simulink model "RRR_with_CTC_task_space"  (Simulink 8.5)
settings: Solver=ode113  StartTime=0.0  StopTime=T_f  RelTol=RT  AbsTol=AT
values from neighbouring files (symbols this model uses):
  kp = x(24)    [PRBDM_3R_CTC.m]    (also in PRBDM_3R_main.m = 20; PRBDM_3R_test001.m = 2; PRBDM_CTC_task.m = z(30); RRR_CTC.m)
  kv = x(23)    [PRBDM_3R_CTC.m]    (also in PRBDM_3R_main.m = 40; PRBDM_3R_test001.m = 4; PRBDM_CTC_task.m = z(29); RRR_CTC.m)
  L1 = z(8)    [Forward_kinematics.m]    (also in GeometricCalculation_simulink.m = Geoparams(5); Jacobi.m = x(4); PRBDM_3R_CTC.m = x(19); PRBDM_3R_Dynamic_Matrices_NewtonEular.m = robot_params(4))
  L2 = z(9)    [Forward_kinematics.m]    (also in GeometricCalculation_simulink.m = Geoparams(6); Jacobi.m = x(5); PRBDM_3R_CTC.m = x(20); PRBDM_3R_Dynamic_Matrices_NewtonEular.m = robot_params(5))
  L3 = z(10)    [Forward_kinematics.m]    (also in GeometricCalculation_simulink.m = Geoparams(7); Jacobi.m = x(6); PRBDM_3R_CTC.m = x(21); PRBDM_3R_Dynamic_Matrices_NewtonEular.m = robot_params(6))
  m1 = x(16)    [PRBDM_3R_CTC.m]    (also in PRBDM_3R_Dynamic_Matrices_NewtonEular.m = robot_params(1); PRBDM_3R_parameters.m = 0.35; PRBDM_3R_parameters.mat = 0.35; PRBDM_3R_test001.m = 0.1)
  m2 = x(17)    [PRBDM_3R_CTC.m]    (also in PRBDM_3R_Dynamic_Matrices_NewtonEular.m = robot_params(2); PRBDM_3R_parameters.m = 0.4; PRBDM_3R_parameters.mat = 0.4; PRBDM_3R_test001.m = 0.1)
  m3 = x(18)    [PRBDM_3R_CTC.m]    (also in PRBDM_3R_Dynamic_Matrices_NewtonEular.m = robot_params(3); PRBDM_3R_parameters.m = 0.15; PRBDM_3R_parameters.mat = 0.15; PRBDM_3R_test001.m = 0.1)
  W = x(22)    [PRBDM_3R_CTC.m]    (also in PRBDM_3R_Dynamic_Matrices_NewtonEular.m = robot_params(7); PRBDM_3R_Dynamics.m = in4dyn(20); PRBDM_3R_Dynamics00.m = in4dyn(20); PRBDM_3R_DynamicsPID.m = in4dyn(20))
settings Model: Creator=sayar  LastModifiedBy=mahdiehbabaiasl
settings DataIOCC: LimitDataPoints=off  SignalLoggingSaveFormat=Dataset  Refine=RF
settings DebuggingCC: SolverPrmCheckMsg=warning  FcnCallInpInsideContextMsg=UseLocalSettings

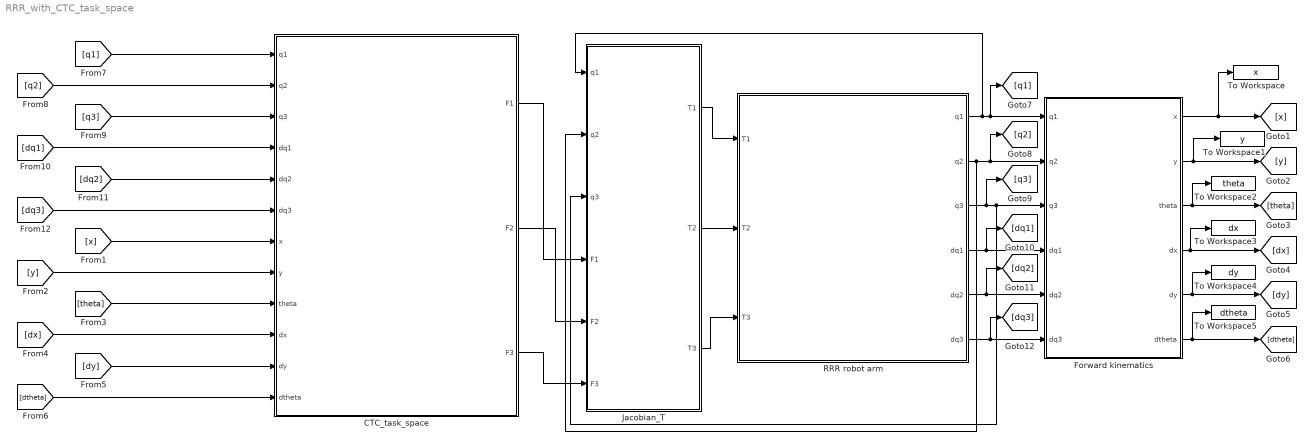
== system RRR_with_CTC_task_space ==
  CTC_task_space : Subsystem
  Forward kinematics : Subsystem
  Jacobian_T : Subsystem
  RRR robot arm : Subsystem
      mask Display: image(imread('RRR.png'))
  To Workspace : ToWorkspace  VariableName=x  SampleTime=-1
  To Workspace1 : ToWorkspace  VariableName=y  SampleTime=-1
  To Workspace2 : ToWorkspace  VariableName=theta  SampleTime=-1
  To Workspace3 : ToWorkspace  VariableName=dx  SampleTime=-1
  To Workspace4 : ToWorkspace  VariableName=dy  SampleTime=-1
  To Workspace5 : ToWorkspace  VariableName=dtheta  SampleTime=-1
  wires:
  [x] -> CTC_task_space/7(x)
  [y] -> CTC_task_space/8(y)
  [theta] -> CTC_task_space/9(theta)
  [dx] -> CTC_task_space/10(dx)
  [dy] -> CTC_task_space/11(dy)
  RRR robot arm/1(q1) -> Jacobian_T/1(q1), [q1], Forward kinematics/1(q1)
  RRR robot arm/2(q2) -> [q2], Forward kinematics/2(q2), Jacobian_T/2(q2)
  RRR robot arm/3(q3) -> [q3], Jacobian_T/3(q3), Forward kinematics/3(q3)
  RRR robot arm/4(dq1) -> [dq1], Forward kinematics/4(dq1)
  RRR robot arm/5(dq2) -> [dq2], Forward kinematics/5(dq2)
  RRR robot arm/6(dq3) -> [dq3], Forward kinematics/6(dq3)
  Forward kinematics/1(x) -> To Workspace/1, [x]
  Forward kinematics/2(y) -> To Workspace1/1, [y]
  Forward kinematics/3(theta) -> To Workspace2/1, [theta]
  Forward kinematics/4(dx) -> To Workspace3/1, [dx]
  Forward kinematics/5(dy) -> To Workspace4/1, [dy]
  Forward kinematics/6(dtheta) -> To Workspace5/1, [dtheta]
  Jacobian_T/1(T1) -> RRR robot arm/1(T1)
  Jacobian_T/2(T2) -> RRR robot arm/2(T2)
  Jacobian_T/3(T3) -> RRR robot arm/3(T3)
  [q1] -> CTC_task_space/1(q1)
  [q2] -> CTC_task_space/2(q2)
  [q3] -> CTC_task_space/3(q3)
  [dq1] -> CTC_task_space/4(dq1)
  [dq2] -> CTC_task_space/5(dq2)
  [dq3] -> CTC_task_space/6(dq3)
  [dtheta] -> CTC_task_space/12(dtheta)
  CTC_task_space/1(F1) -> Jacobian_T/4(F1)
  CTC_task_space/2(F2) -> Jacobian_T/5(F2)
  CTC_task_space/3(F3) -> Jacobian_T/6(F3)

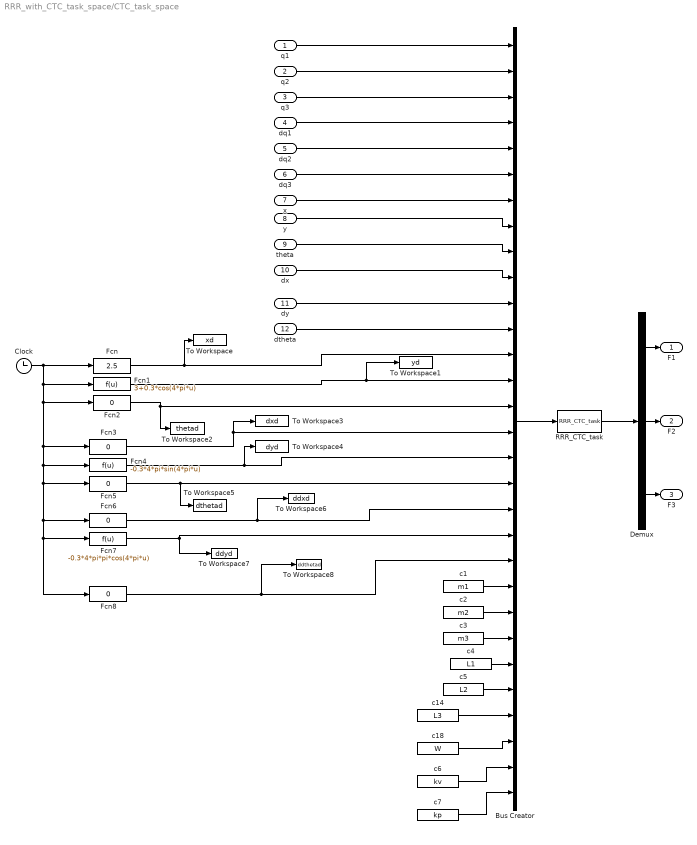
== system RRR_with_CTC_task_space/CTC_task_space ==
  q1 : Inport
  q2 : Inport  Port=2
  q3 : Inport  Port=3
  dq1 : Inport  Port=4
  dq2 : Inport  Port=5
  dq3 : Inport  Port=6
  x : Inport  Port=7
  y : Inport  Port=8
  theta : Inport  Port=9
  dx : Inport  Port=10
  dy : Inport  Port=11
  dtheta : Inport  Port=12
  Bus Creator : BusCreator  Inputs=30
  Clock : Clock
  Demux : Demux  Outputs=3
  Fcn : Fcn  Expr=2.5
  Fcn1 : Fcn  Expr=3+0.3*cos(4*pi*u)
  Fcn{2..3,5..6,8} (5 alike) : Fcn  Expr=0
  Fcn4 : Fcn  Expr=-0.3*4*pi*sin(4*pi*u)
  Fcn7 : Fcn  Expr=-0.3*4*pi*pi*cos(4*pi*u)
  RRR_CTC_task : MATLABFcn  MATLABFcn=RRR_CTC_task  OutputDimensions=3
  To Workspace : ToWorkspace  VariableName=xd  SampleTime=-1
  To Workspace1 : ToWorkspace  VariableName=yd  SampleTime=-1
  To Workspace2 : ToWorkspace  VariableName=thetad  SampleTime=-1
  To Workspace3 : ToWorkspace  VariableName=dxd  SampleTime=-1
  To Workspace4 : ToWorkspace  VariableName=dyd  SampleTime=-1
  To Workspace5 : ToWorkspace  VariableName=dthetad  SampleTime=-1
  To Workspace6 : ToWorkspace  VariableName=ddxd  SampleTime=-1
  To Workspace7 : ToWorkspace  VariableName=ddyd  SampleTime=-1
  To Workspace8 : ToWorkspace  VariableName=ddthetad  SampleTime=-1
  c1 : Constant  Value=m1
  c14 : Constant  Value=L3
  c18 : Constant  Value=W
  c2 : Constant  Value=m2
  c3 : Constant  Value=m3
  c4 : Constant  Value=L1
  c5 : Constant  Value=L2
  c6 : Constant  Value=kv
  c7 : Constant  Value=kp
  F1 : Outport
  F2 : Outport  Port=2
  F3 : Outport  Port=3
  wires:
  q3/1 -> Bus Creator/3
  RRR_CTC_task/1 -> Demux/1
  q1/1 -> Bus Creator/1
  Demux/3 -> F3/1
  q2/1 -> Bus Creator/2
  dq2/1 -> Bus Creator/5
  dq1/1 -> Bus Creator/4
  Demux/2 -> F2/1
  dq3/1 -> Bus Creator/6
  Demux/1 -> F1/1
  Bus Creator/1 -> RRR_CTC_task/1
  Clock/1 -> Fcn5/1, Fcn8/1, Fcn7/1, Fcn6/1, Fcn4/1, Fcn3/1, Fcn2/1, Fcn1/1, Fcn/1
  Fcn2/1 -> Bus Creator/15, To Workspace2/1
  Fcn3/1 -> Bus Creator/16, To Workspace3/1
  Fcn6/1 -> Bus Creator/19, To Workspace6/1
  Fcn7/1 -> To Workspace7/1, Bus Creator/20
  x/1 -> Bus Creator/7
  y/1 -> Bus Creator/8
  theta/1 -> Bus Creator/9
  dx/1 -> Bus Creator/10
  dy/1 -> Bus Creator/11
  dtheta/1 -> Bus Creator/12
  Fcn5/1 -> Bus Creator/18, To Workspace5/1
  Fcn/1 -> To Workspace/1, Bus Creator/13
  Fcn1/1 -> To Workspace1/1, Bus Creator/14
  Fcn4/1 -> Bus Creator/17, To Workspace4/1
  Fcn8/1 -> To Workspace8/1, Bus Creator/21
  c1/1 -> Bus Creator/22
  c2/1 -> Bus Creator/23
  c3/1 -> Bus Creator/24
  c4/1 -> Bus Creator/25
  c5/1 -> Bus Creator/26
  c14/1 -> Bus Creator/27
  c18/1 -> Bus Creator/28
  c6/1 -> Bus Creator/29
  c7/1 -> Bus Creator/30

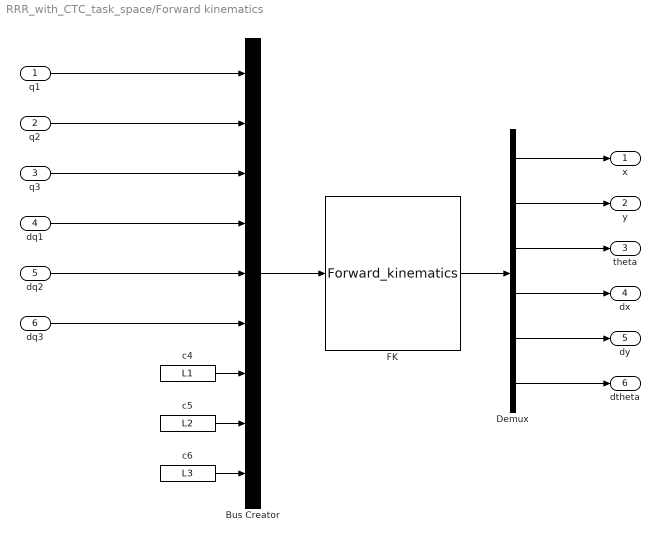
== system RRR_with_CTC_task_space/Forward kinematics ==
  q1 : Inport
  q2 : Inport  Port=2
  q3 : Inport  Port=3
  dq1 : Inport  Port=4
  dq2 : Inport  Port=5
  dq3 : Inport  Port=6
  Bus Creator : BusCreator  Inputs=9
  Demux : Demux  Outputs=6
  FK : MATLABFcn  MATLABFcn=Forward_kinematics  OutputDimensions=6
  c4 : Constant  Value=L1
  c5 : Constant  Value=L2
  c6 : Constant  Value=L3
  x : Outport
  y : Outport  Port=2
  theta : Outport  Port=3
  dx : Outport  Port=4
  dy : Outport  Port=5
  dtheta : Outport  Port=6
  wires:
  c6/1 -> Bus Creator/9
  Demux/1 -> x/1
  Demux/4 -> dx/1
  c4/1 -> Bus Creator/7
  Demux/5 -> dy/1
  q2/1 -> Bus Creator/2
  q1/1 -> Bus Creator/1
  q3/1 -> Bus Creator/3
  Bus Creator/1 -> FK/1
  dq2/1 -> Bus Creator/5
  Demux/2 -> y/1
  FK/1 -> Demux/1
  dq1/1 -> Bus Creator/4
  Demux/3 -> theta/1
  dq3/1 -> Bus Creator/6
  Demux/6 -> dtheta/1
  c5/1 -> Bus Creator/8

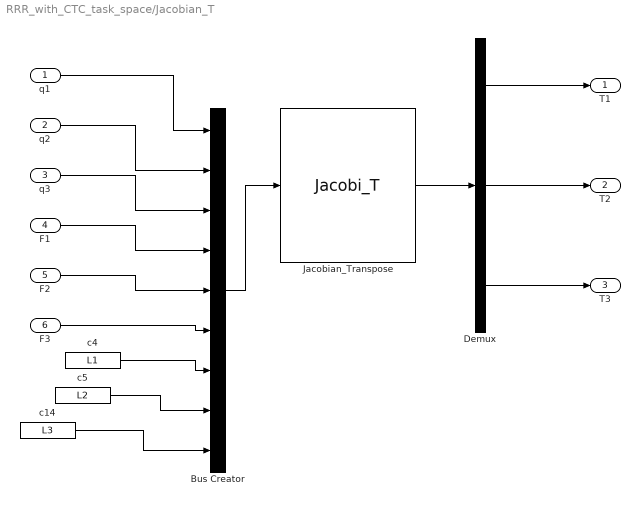
== system RRR_with_CTC_task_space/Jacobian_T ==
  q1 : Inport
  q2 : Inport  Port=2
  q3 : Inport  Port=3
  F1 : Inport  Port=4
  F2 : Inport  Port=5
  F3 : Inport  Port=6
  Bus Creator : BusCreator  Inputs=9
  Demux : Demux  Outputs=3
  Jacobian_Transpose : MATLABFcn  MATLABFcn=Jacobi_T  OutputDimensions=3
  c14 : Constant  Value=L3
  c4 : Constant  Value=L1
  c5 : Constant  Value=L2
  T1 : Outport
  T2 : Outport  Port=2
  T3 : Outport  Port=3
  wires:
  Jacobian_Transpose/1 -> Demux/1
  Demux/2 -> T2/1
  Bus Creator/1 -> Jacobian_Transpose/1
  Demux/1 -> T1/1
  Demux/3 -> T3/1
  F1/1 -> Bus Creator/4
  F2/1 -> Bus Creator/5
  F3/1 -> Bus Creator/6
  q1/1 -> Bus Creator/1
  q2/1 -> Bus Creator/2
  q3/1 -> Bus Creator/3
  c5/1 -> Bus Creator/8
  c14/1 -> Bus Creator/9
  c4/1 -> Bus Creator/7

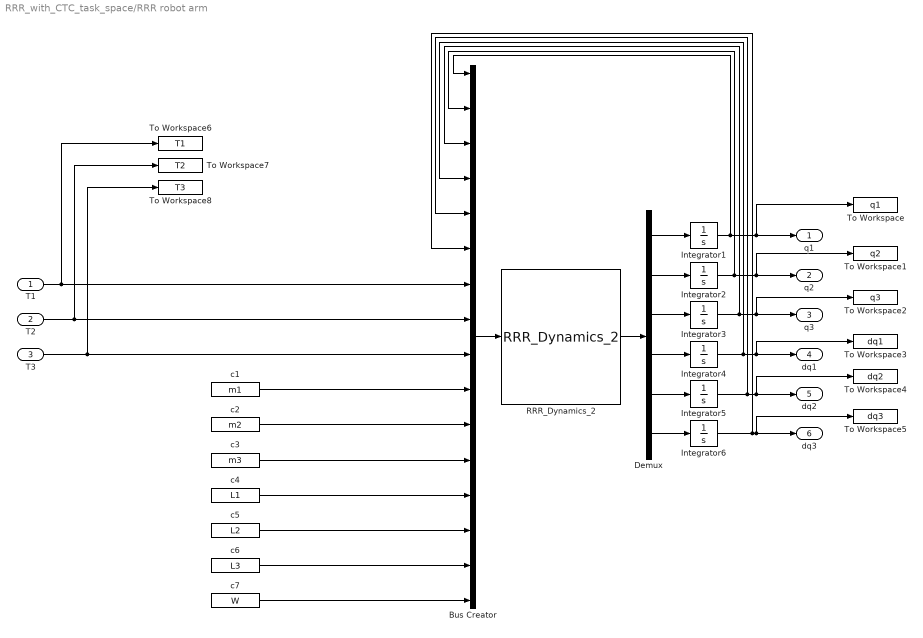
== system RRR_with_CTC_task_space/RRR robot arm ==
  T1 : Inport
  T2 : Inport  Port=2
  T3 : Inport  Port=3
  Bus Creator : BusCreator  Inputs=16
  Demux : Demux  Outputs=6
  Integrator{1,4..6} (4 alike) : Integrator
  Integrator2 : Integrator  InitialCondition=3*pi/4
  Integrator3 : Integrator  InitialCondition=-3*pi/4
  RRR_Dynamics_2 : MATLABFcn  MATLABFcn=RRR_Dynamics_2  OutputDimensions=6
  To Workspace : ToWorkspace  VariableName=q1  SampleTime=-1
  To Workspace1 : ToWorkspace  VariableName=q2  SampleTime=-1
  To Workspace2 : ToWorkspace  VariableName=q3  SampleTime=-1
  To Workspace3 : ToWorkspace  VariableName=dq1  SampleTime=-1
  To Workspace4 : ToWorkspace  VariableName=dq2  SampleTime=-1
  To Workspace5 : ToWorkspace  VariableName=dq3  SampleTime=-1
  To Workspace6 : ToWorkspace  VariableName=T1  SampleTime=-1
  To Workspace7 : ToWorkspace  VariableName=T2  SampleTime=-1
  To Workspace8 : ToWorkspace  VariableName=T3  SampleTime=-1
  c1 : Constant  Value=m1
  c2 : Constant  Value=m2
  c3 : Constant  Value=m3
  c4 : Constant  Value=L1
  c5 : Constant  Value=L2
  c6 : Constant  Value=L3
  c7 : Constant  Value=W
  q1 : Outport
  q2 : Outport  Port=2
  q3 : Outport  Port=3
  dq1 : Outport  Port=4
  dq2 : Outport  Port=5
  dq3 : Outport  Port=6
  wires:
  Demux/1 -> Integrator1/1
  Demux/2 -> Integrator2/1
  Demux/3 -> Integrator3/1
  Demux/4 -> Integrator4/1
  Demux/5 -> Integrator5/1
  Demux/6 -> Integrator6/1
  Integrator1/1 -> Bus Creator/1, q1/1, To Workspace/1
  Integrator2/1 -> Bus Creator/2, q2/1, To Workspace1/1
  Integrator3/1 -> Bus Creator/3, q3/1, To Workspace2/1
  Integrator4/1 -> Bus Creator/4, dq1/1, To Workspace3/1
  Integrator5/1 -> Bus Creator/5, dq2/1, To Workspace4/1
  Integrator6/1 -> Bus Creator/6, dq3/1, To Workspace5/1
  c1/1 -> Bus Creator/10
  c2/1 -> Bus Creator/11
  RRR_Dynamics_2/1 -> Demux/1
  Bus Creator/1 -> RRR_Dynamics_2/1
  T3/1 -> To Workspace8/1, Bus Creator/9
  T2/1 -> To Workspace7/1, Bus Creator/8
  T1/1 -> To Workspace6/1, Bus Creator/7
  c3/1 -> Bus Creator/12
  c4/1 -> Bus Creator/13
  c5/1 -> Bus Creator/14
  c6/1 -> Bus Creator/15
  c7/1 -> Bus Creator/16
